simulink model "simulinkDraw"  (R2024a)
settings: Solver=VariableStepAuto  StartTime=0.0  StopTime=10.0  RelTol=1e-3
settings Model: Creator=vinicius.rocha-miran  LastModifiedBy=vinicius.rocha-miran

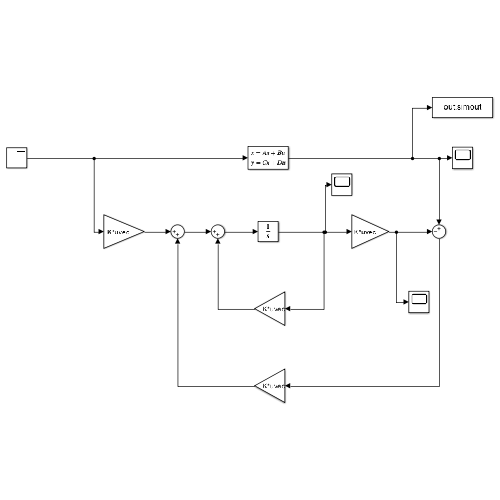
[thumbnail: Simulink's stored preview of the top-level diagram]
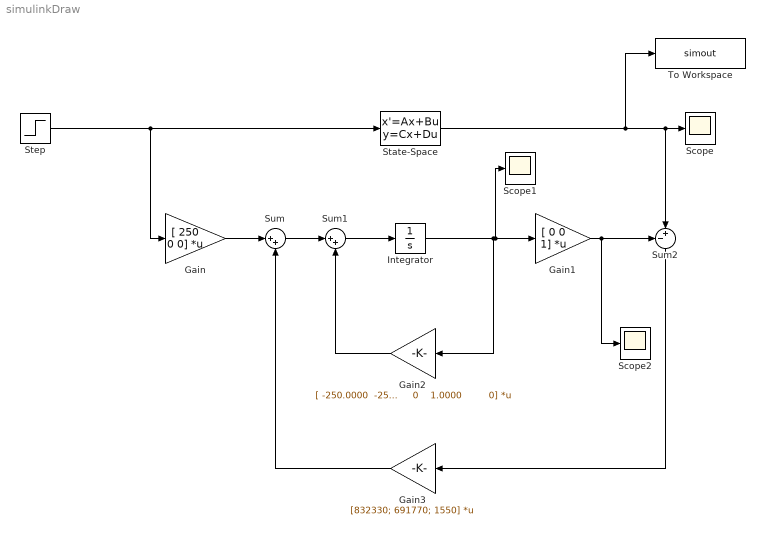
== system simulinkDraw ==
  Gain : Gain  Gain=|  Multiplication=Matrix(K*u) (u vector)
      | [   250
      |      0
      |      0]
  Gain1 : Gain  Gain="[     0     0     1]"  Multiplication=Matrix(K*u) (u vector)
  Gain2 : Gain  Gain=|  Multiplication=Matrix(K*u) (u vector)
      | [ -250.0000  -25.0000         0
      |    50.0000   -1.5000         0
      |          0    1.0000         0]
  Gain3 : Gain  Gain=[832330; 691770; 1550]  Multiplication=Matrix(K*u) (u vector)
  Integrator : Integrator
  Scope : Scope
  Scope1 : Scope
  Scope2 : Scope
  State-Space : StateSpace  A=|  B=|  C="[     0     0     1]"  D=0  InitialCondition=[0.01;0.02;0.03]
      A=|
      | [-250.00 -25.00 0; 50.00 -1.50 0;
      | 0 1.00 0]
      B=|
      | [
      |    250;
      |      0;
      |      0]
  Step : Step  Before=1  SampleTime=0
  Sum : Sum  Inputs=|++
  Sum1 : Sum  Inputs=|++
  Sum2 : Sum  Inputs=-+|
  To Workspace : ToWorkspace  VariableName=simout  SaveFormat=Timeseries  SampleTime=-1
  wires:
  Step/1 -> Gain/1, State-Space/1
  State-Space/1 -> To Workspace/1, Sum2/2, Scope/1
  Integrator/1 -> Gain2/1, Scope1/1, Gain1/1
  Sum1/1 -> Integrator/1
  Sum/1 -> Sum1/1
  Gain/1 -> Sum/1
  Gain2/1 -> Sum1/2
  Gain3/1 -> Sum/2
  Gain1/1 -> Scope2/1, Sum2/1
  Sum2/1 -> Gain3/1
